simulink model "feedback"  (R2018a)
settings: Solver=ode45  StartTime=0.0  StopTime=3  FixedStep=0.01  RelTol=1e-3  EnableMultiTasking=on
InitFcn:
  | Ts=1e-6
undefined symbols (not defined in the file): DiscIntNeverNeededParam
libraries: powerlib x9, simulink x1
settings Model: Creator=Omar.Hazem  LastModifiedBy=Omar.Hazem
settings SolverCC: AlgebraicLoopSolver=LineSearch
settings DataIOCC: LimitDataPoints=on  SaveFormat=Array
settings OptimizationCC: LifeSpan=inf
settings DebuggingCC: MaxConsecutiveZCsMsg=none  SolverPrmCheckMsg=warning  SFUnexpectedBacktrackingDiag=warning  SFNoUnconditionalDefaultTransitionDiag=warning  SFExecutionAtInitializationDiag=none
settings HardwareCC: ProdBitPerPointer=32  ProdBitPerSizeT=32  ProdBitPerPtrDiffT=32  ProdLargestAtomicFloat=None  ProdIntDivRoundTo=Undefined  ProdEndianess=Unspecified  ProdWordSize=32  ProdHWDeviceType=32-bit Generic
settings ModelReferenceCC: PropagateSignalLabelsOutOfModel=off
settings CodeAppCC: StateflowObjectComments=on
settings GRTTargetCC: TargetLangStandard=C89/C90 (ANSI)  GeneratePreprocessorConditionals=Disable all
settings ConfigComp: CovMetricSettings=dw  CovHtmlReporting=on  CovSaveCumulativeToWorkspaceVar=on  CovSaveSingleToWorkspaceVar=on  CovExternalEMLEnable=off  CovSFcnEnable=off
settings SimscapeCC: SimscapeNormalizeSystem=off

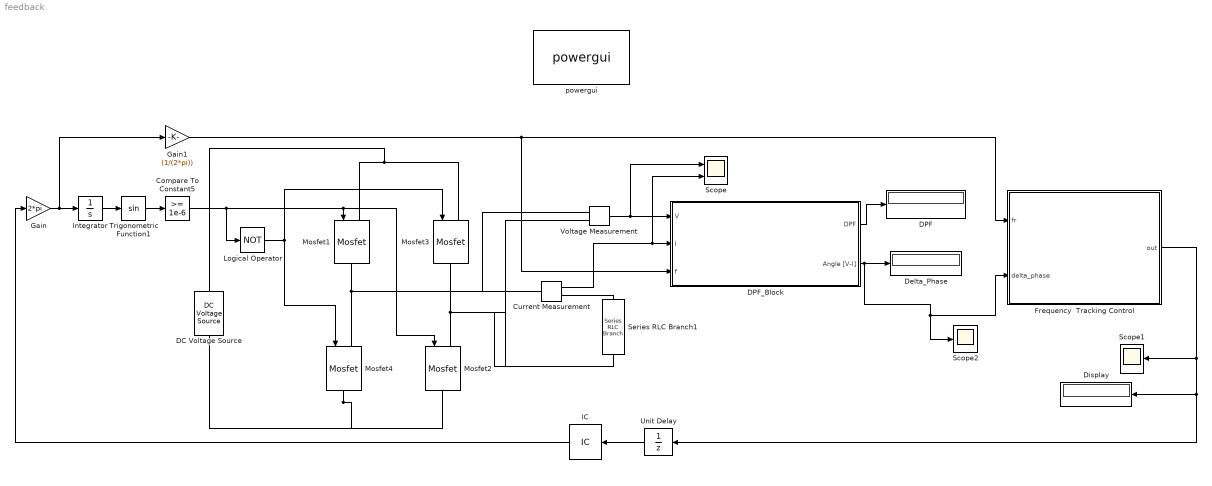
== system feedback ==
  Compare To Constant5 : simulink/Logic and Bit Operations/Compare To Constant  relop=>=  const=1e-6  OutDataTypeStr=boolean  ZeroCross=off
  Current Measurement : powerlib/Measurements/Current Measurement  PhasorSimulation=off  OutputType=Complex  PSBequivalent=0
  DC Voltage Source : powerlib/Electrical Sources/DC Voltage Source  Amplitude=100  Measurements=None
  DPF : Display
  DPF_Block : Subsystem
  Delta_Phase : Display
  Display : Display
  Frequency  Tracking Control : MATLAB Function  TreatAsAtomicUnit=on
  Gain : Gain  Gain=2*pi
  Gain1 : Gain  Gain=(1/(2*pi))
  IC : InitialCondition  Value=35000
  Integrator : Integrator
  Logical Operator : Logic  Operator=NOT  AllPortsSameDT=off  OutDataTypeStr=boolean
  Mosfet{1..4} (4 alike) : powerlib/Power Electronics/Mosfet  Ron=0.1  Lon=0  Rd=0.01  Vfd=0  IC=0  Rs=1e5  Cs=inf  Measurements=off
  Scope : Scope  NumInputPorts=2
  Scope1 : Scope
  Scope2 : Scope
  Series RLC Branch1 : powerlib/Elements/Series RLC Branch  LConnTagsString=__new0  RConnTagsString=__new0  BranchType=RLC  Resistance=30  Inductance=1e-3  SetiL0=off  InitialCurrent=0  Capacitance=16e-9  Setx0=off  InitialVoltage=0  Measurements=None
  Trigonometric Function1 : Trigonometry
  Unit Delay : UnitDelay  SampleTime=-1
  Voltage Measurement : powerlib/Measurements/Voltage Measurement  PhasorSimulation=off  OutputType=Complex  PSBequivalent=0
  powergui : powerlib/powergui  Priority=1  SimulationMode=Continuous  SampleTime=50e-6  frequency=1  Iterations=50  frequencyindice=0  Pbase=100e6  ErrMax=1e-4  UnitsV=kV  UnitsW=MW  buscounter=0  FunctionMessages=off  echomessages=off  EnableUseOfTLC=off  CurrentSourceSwitches=on  DisableSnubberDevices=off  DisableRonSwitches=off  DisableVfSwitches=off  DisplayEquations=off  SolverType=Tustin  Interpol=off  ExternalGateDelay=off  methode=off  Ts=0  x0status=blocks  SPID=off  SwTol=0  HookPort=off  RestoreLinks=warning  ResistiveCurrentMeasurement=off  Frange=[0:2:500]  Ylog=off  Xlog=on  ShowGrid=off  save=off  variable=ZData  structure=0  ZoomFFT=off  StartTime=0.0  cycles=1  DisplayStyle=1  fundamental=60  FreqAxis=off  MaxFrequency=1000  frequencyindicesteady=1  RmsSteady=1  display=off
  wires:
  Compare To Constant5/1 -> Mosfet2/1, Mosfet1/1, Logical Operator/1
  Logical Operator/1 -> Mosfet3/1, Mosfet4/1
  Integrator/1 -> Trigonometric Function1/1
  Trigonometric Function1/1 -> Compare To Constant5/1
  DPF_Block/2(Angle [V-I]) -> Scope2/1, Frequency  Tracking Control/2(delta_phase), Delta_Phase/1
  DPF_Block/1(DPF) -> DPF/1
  Voltage Measurement/1 -> Scope/1, DPF_Block/1(V)
  Gain/1 -> Integrator/1, Gain1/1
  Gain1/1 -> Frequency  Tracking Control/1(fr), DPF_Block/3(f)
  Unit Delay/1 -> IC/1
  IC/1 -> Gain/1
  Current Measurement/1 -> DPF_Block/2(I), Scope/2
  Frequency  Tracking Control/1(out) -> Display/1, Unit Delay/1, Scope1/1
  connections:
  Mosfet1/RConn1 -- Voltage Measurement/LConn1 -- Current Measurement/LConn1 -- Mosfet4/LConn1
  Mosfet1/LConn1 -- Mosfet3/LConn1 -- DC Voltage Source/RConn1
  Mosfet2/LConn1 -- Series RLC Branch1/RConn1 -- Voltage Measurement/LConn2 -- Mosfet3/RConn1
  Mosfet4/RConn1 -- Mosfet2/RConn1 -- DC Voltage Source/LConn1
  Current Measurement/RConn1 -- Series RLC Branch1/LConn1

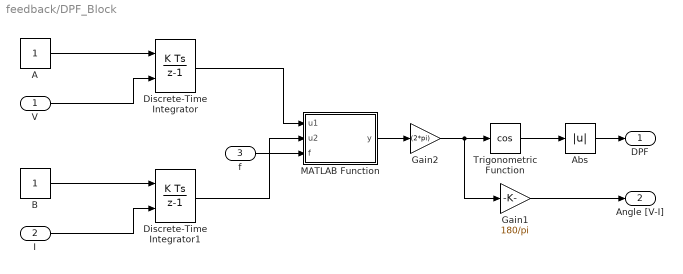
== system feedback/DPF_Block ==
  V : Inport
  I : Inport  Port=2
  f : Inport  Port=3
  A : Constant
  Abs : Abs
  B : Constant
  Discrete-Time Integrator : DiscreteIntegrator  ExternalReset=rising  SampleTime=Ts  ICPrevOutput=DiscIntNeverNeededParam  ICPrevScaledInput=DiscIntNeverNeededParam
  Discrete-Time Integrator1 : DiscreteIntegrator  ExternalReset=rising  SampleTime=Ts  ICPrevOutput=DiscIntNeverNeededParam  ICPrevScaledInput=DiscIntNeverNeededParam
  Gain1 : Gain  Gain=180/pi
  Gain2 : Gain  Gain=(2*pi)
  MATLAB Function : MATLAB Function  TreatAsAtomicUnit=on
  Trigonometric Function : Trigonometry  Operator=cos
  DPF : Outport
  Angle [V-I] : Outport  Port=2
  wires:
  I/1 -> Discrete-Time Integrator1/2
  V/1 -> Discrete-Time Integrator/2
  A/1 -> Discrete-Time Integrator/1
  B/1 -> Discrete-Time Integrator1/1
  Discrete-Time Integrator1/1 -> MATLAB Function/2(u2)
  Trigonometric Function/1 -> Abs/1
  Discrete-Time Integrator/1 -> MATLAB Function/1(u1)
  Abs/1 -> DPF/1
  Gain1/1 -> Angle [V-I]/1
  f/1 -> MATLAB Function/3(f)
  MATLAB Function/1(y) -> Gain2/1
  Gain2/1 -> Gain1/1, Trigonometric Function/1

== matlab function feedback/Frequency  Tracking Control ==
  data: fr input; delta_phase input; out output
function out = correct(fr, delta_phase)
step = 0.005;
initcond = 35000;
perfect = 0;

   if perfect == 0 
       
if (delta_phase > 0)
    out=fr+step;
    
elseif  (delta_phase < 0)
        out=fr-step;  
        
elseif delta_phase == 0
    perfect = fr;
    out = perfect;
else 
    
    out = initcond;
end

   else        
       out = perfect;
   end

== matlab function feedback/DPF_Block/MATLAB Function ==
  data: u1 input; y output; u2 input; f input
function y = fcn(u1, u2, f)
if (u2-u1) > 1/(2*f)
    y = -((1/f + (u1-u2))*f);
elseif (u1-u2) > 1/(2*f)
         y = ((1/f - (u1-u2))*f);
else
    y = -((u1-u2)*f);
end
